simulink library "environment"  (R2024a)
settings: Solver=VariableStepAuto  StartTime=0.0  StopTime=10.0  RelTol=1e-3
undefined symbols (not defined in the file or in its folder): Heigth_brick, Heigth_ramp, Heigth_wall, Length_brick, Length_ramp, Length_wall, theta, Wall1, Wall2, Wall3, Wall4, Wall5, Wall6, Width_brick, Width_ramp, Width_wall, X, Y, Z
libraries: sm_lib x81, nesl_utility x28, $bdroot x5
(part 2 of 2)

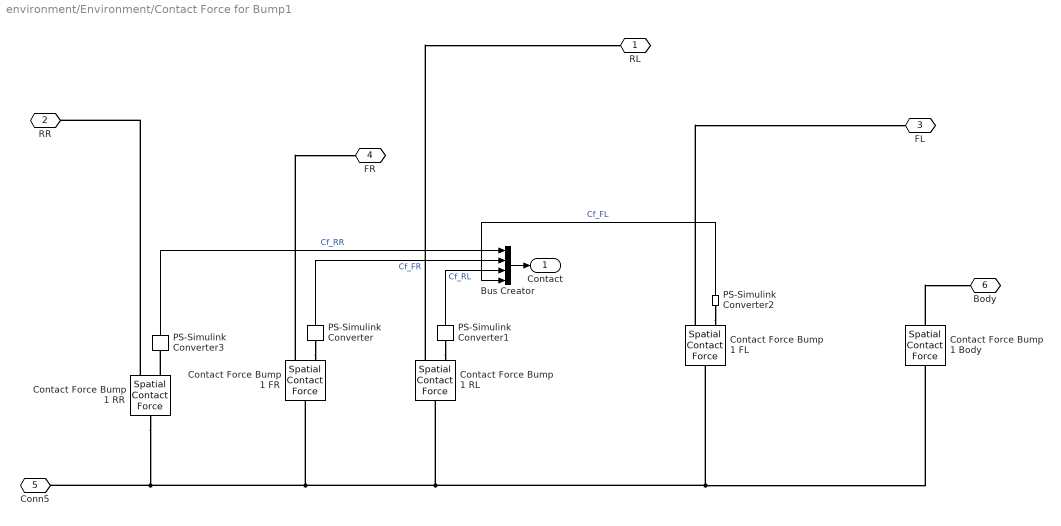
== system environment/Environment/Contact Force for Bump1 ==
  Bus Creator : BusCreator  Inputs=4
  Contact Force Bump 1 Body : sm_lib/Forces and Torques/Spatial Contact Force  NormalForceType=SmoothSpringDamper  NormalStiffness=Stiffnesscoefficient  NormalStiffnessUnits=N/m  NormalDamping=Damping_Factor  NormalDampingUnits=N/(m/s)  NormalTransitionRegionWidth=Transition_Region_Width  NormalTransitionRegionWidthUnits=m  FrictionType=SmoothStickSlip  CoefficientOfStaticFriction=Static_Friction  CoefficientOfDynamicFriction=Dynamic_Friction  FrictionalCriticalVelocity=Critical_Velocity  FrictionalCriticalVelocityUnits=m/s  SenseContactSignal=off  SensePenetrationDepth=off  SenseSeparationDistance=off  SenseNormalForceMagnitude=off  SenseFrictionalForceMagnitude=off  SenseNormalVelocity=off  SenseTangentialVelocity=off  SenseContactBaseRotation=off  SenseContactBaseTranslation=off  SenseContactFollowerRotation=off  SenseContactFollowerTranslation=off  ZeroCrossDetectContactStartAndEnd=off
  Contact Force Bump 1 FL : sm_lib/Forces and Torques/Spatial Contact Force  NormalForceType=SmoothSpringDamper  NormalStiffness=Stiffnesscoefficient  NormalStiffnessUnits=N/m  NormalDamping=Damping_Factor  NormalDampingUnits=N/(m/s)  NormalTransitionRegionWidth=Transition_Region_Width  NormalTransitionRegionWidthUnits=m  FrictionType=SmoothStickSlip  CoefficientOfStaticFriction=Static_Friction  CoefficientOfDynamicFriction=Dynamic_Friction  FrictionalCriticalVelocity=Critical_Velocity  FrictionalCriticalVelocityUnits=m/s  SenseContactSignal=off  SensePenetrationDepth=off  SenseSeparationDistance=off  SenseNormalForceMagnitude=on  SenseFrictionalForceMagnitude=off  SenseNormalVelocity=off  SenseTangentialVelocity=off  SenseContactBaseRotation=off  SenseContactBaseTranslation=off  SenseContactFollowerRotation=off  SenseContactFollowerTranslation=off  ZeroCrossDetectContactStartAndEnd=off
  Contact Force Bump 1 FR : sm_lib/Forces and Torques/Spatial Contact Force  NormalForceType=SmoothSpringDamper  NormalStiffness=Stiffnesscoefficient  NormalStiffnessUnits=N/m  NormalDamping=Damping_Factor  NormalDampingUnits=N/(m/s)  NormalTransitionRegionWidth=Transition_Region_Width  NormalTransitionRegionWidthUnits=m  FrictionType=SmoothStickSlip  CoefficientOfStaticFriction=Static_Friction  CoefficientOfDynamicFriction=Dynamic_Friction  FrictionalCriticalVelocity=Critical_Velocity  FrictionalCriticalVelocityUnits=m/s  SenseContactSignal=off  SensePenetrationDepth=off  SenseSeparationDistance=off  SenseNormalForceMagnitude=on  SenseFrictionalForceMagnitude=off  SenseNormalVelocity=off  SenseTangentialVelocity=off  SenseContactBaseRotation=off  SenseContactBaseTranslation=off  SenseContactFollowerRotation=off  SenseContactFollowerTranslation=off  ZeroCrossDetectContactStartAndEnd=off
  Contact Force Bump 1 RL : sm_lib/Forces and Torques/Spatial Contact Force  NormalForceType=SmoothSpringDamper  NormalStiffness=Stiffnesscoefficient  NormalStiffnessUnits=N/m  NormalDamping=Damping_Factor  NormalDampingUnits=N/(m/s)  NormalTransitionRegionWidth=Transition_Region_Width  NormalTransitionRegionWidthUnits=m  FrictionType=SmoothStickSlip  CoefficientOfStaticFriction=Static_Friction  CoefficientOfDynamicFriction=Dynamic_Friction  FrictionalCriticalVelocity=Critical_Velocity  FrictionalCriticalVelocityUnits=m/s  SenseContactSignal=off  SensePenetrationDepth=off  SenseSeparationDistance=off  SenseNormalForceMagnitude=on  SenseFrictionalForceMagnitude=off  SenseNormalVelocity=off  SenseTangentialVelocity=off  SenseContactBaseRotation=off  SenseContactBaseTranslation=off  SenseContactFollowerRotation=off  SenseContactFollowerTranslation=off  ZeroCrossDetectContactStartAndEnd=off
  Contact Force Bump 1 RR : sm_lib/Forces and Torques/Spatial Contact Force  NormalForceType=SmoothSpringDamper  NormalStiffness=Stiffnesscoefficient  NormalStiffnessUnits=N/m  NormalDamping=Damping_Factor  NormalDampingUnits=N/(m/s)  NormalTransitionRegionWidth=Transition_Region_Width  NormalTransitionRegionWidthUnits=m  FrictionType=SmoothStickSlip  CoefficientOfStaticFriction=Static_Friction  CoefficientOfDynamicFriction=Dynamic_Friction  FrictionalCriticalVelocity=Critical_Velocity  FrictionalCriticalVelocityUnits=m/s  SenseContactSignal=off  SensePenetrationDepth=off  SenseSeparationDistance=off  SenseNormalForceMagnitude=on  SenseFrictionalForceMagnitude=off  SenseNormalVelocity=off  SenseTangentialVelocity=off  SenseContactBaseRotation=off  SenseContactBaseTranslation=off  SenseContactFollowerRotation=off  SenseContactFollowerTranslation=off  ZeroCrossDetectContactStartAndEnd=off
  PS-Simulink Converter{,1..3} (4 alike) : nesl_utility/PS-Simulink Converter  PhysicalDomain=network_engine_domain  SubClassName=ps_output  LeftPortType=input  RightPortType=output  PseudoPeriodic=off  Frequencies=[]  VectorFormat=inherit  Unit=inherit  AffineConversion=off
  RL : PMIOPort  Side=Right
  RR : PMIOPort  Port=2  Side=Right
  FL : PMIOPort  Port=3  Side=Right
  FR : PMIOPort  Port=4  Side=Right
  Conn5 : PMIOPort  Port=5  Side=Left
  Body : PMIOPort  Port=6  Side=Right
  Contact : Outport
  wires:
  PS-Simulink Converter3/1 -> Bus Creator/1  "Cf_RR"
  PS-Simulink Converter/1 -> Bus Creator/2  "Cf_FR"
  PS-Simulink Converter1/1 -> Bus Creator/3  "Cf_RL"
  PS-Simulink Converter2/1 -> Bus Creator/4  "Cf_FL"
  Bus Creator/1 -> Contact/1
  connections:
  Contact Force Bump 1 RL/LConn1 -- Contact Force Bump 1 FR/LConn1 -- Contact Force Bump 1 RR/LConn1 -- Conn5/RConn1 -- Contact Force Bump 1 FL/LConn1 -- Contact Force Bump 1 Body/LConn1
  Contact Force Bump 1 FR/RConn1 -- FR/RConn1
  Contact Force Bump 1 RL/RConn1 -- RL/RConn1
  Contact Force Bump 1 RR/RConn1 -- RR/RConn1
  Contact Force Bump 1 FL/RConn1 -- FL/RConn1
  Contact Force Bump 1 Body/RConn1 -- Body/RConn1
  PS-Simulink Converter/LConn1 -- Contact Force Bump 1 FR/RConn2
  PS-Simulink Converter1/LConn1 -- Contact Force Bump 1 RL/RConn2
  PS-Simulink Converter2/LConn1 -- Contact Force Bump 1 FL/RConn2
  Contact Force Bump 1 RR/RConn2 -- PS-Simulink Converter3/LConn1

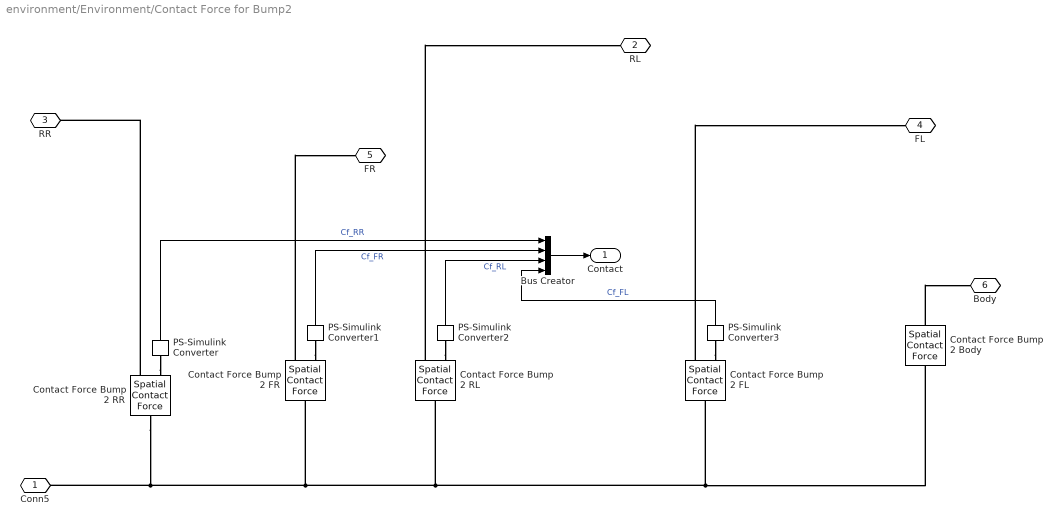
== system environment/Environment/Contact Force for Bump2 ==
  Bus Creator : BusCreator  Inputs=4
  Contact Force Bump 2 Body : sm_lib/Forces and Torques/Spatial Contact Force  NormalForceType=SmoothSpringDamper  NormalStiffness=Stiffnesscoefficient  NormalStiffnessUnits=N/m  NormalDamping=Damping_Factor  NormalDampingUnits=N/(m/s)  NormalTransitionRegionWidth=Transition_Region_Width  NormalTransitionRegionWidthUnits=m  FrictionType=SmoothStickSlip  CoefficientOfStaticFriction=Static_Friction  CoefficientOfDynamicFriction=Dynamic_Friction  FrictionalCriticalVelocity=Critical_Velocity  FrictionalCriticalVelocityUnits=m/s  SenseContactSignal=off  SensePenetrationDepth=off  SenseSeparationDistance=off  SenseNormalForceMagnitude=off  SenseFrictionalForceMagnitude=off  SenseNormalVelocity=off  SenseTangentialVelocity=off  SenseContactBaseRotation=off  SenseContactBaseTranslation=off  SenseContactFollowerRotation=off  SenseContactFollowerTranslation=off  ZeroCrossDetectContactStartAndEnd=off
  Contact Force Bump 2 FL : sm_lib/Forces and Torques/Spatial Contact Force  NormalForceType=SmoothSpringDamper  NormalStiffness=Stiffnesscoefficient  NormalStiffnessUnits=N/m  NormalDamping=Damping_Factor  NormalDampingUnits=N/(m/s)  NormalTransitionRegionWidth=Transition_Region_Width  NormalTransitionRegionWidthUnits=m  FrictionType=SmoothStickSlip  CoefficientOfStaticFriction=Static_Friction  CoefficientOfDynamicFriction=Dynamic_Friction  FrictionalCriticalVelocity=Critical_Velocity  FrictionalCriticalVelocityUnits=m/s  SenseContactSignal=off  SensePenetrationDepth=off  SenseSeparationDistance=off  SenseNormalForceMagnitude=on  SenseFrictionalForceMagnitude=off  SenseNormalVelocity=off  SenseTangentialVelocity=off  SenseContactBaseRotation=off  SenseContactBaseTranslation=off  SenseContactFollowerRotation=off  SenseContactFollowerTranslation=off  ZeroCrossDetectContactStartAndEnd=off
  Contact Force Bump 2 FR : sm_lib/Forces and Torques/Spatial Contact Force  NormalForceType=SmoothSpringDamper  NormalStiffness=Stiffnesscoefficient  NormalStiffnessUnits=N/m  NormalDamping=Damping_Factor  NormalDampingUnits=N/(m/s)  NormalTransitionRegionWidth=Transition_Region_Width  NormalTransitionRegionWidthUnits=m  FrictionType=SmoothStickSlip  CoefficientOfStaticFriction=Static_Friction  CoefficientOfDynamicFriction=Dynamic_Friction  FrictionalCriticalVelocity=Critical_Velocity  FrictionalCriticalVelocityUnits=m/s  SenseContactSignal=off  SensePenetrationDepth=off  SenseSeparationDistance=off  SenseNormalForceMagnitude=on  SenseFrictionalForceMagnitude=off  SenseNormalVelocity=off  SenseTangentialVelocity=off  SenseContactBaseRotation=off  SenseContactBaseTranslation=off  SenseContactFollowerRotation=off  SenseContactFollowerTranslation=off  ZeroCrossDetectContactStartAndEnd=off
  Contact Force Bump 2 RL : sm_lib/Forces and Torques/Spatial Contact Force  NormalForceType=SmoothSpringDamper  NormalStiffness=Stiffnesscoefficient  NormalStiffnessUnits=N/m  NormalDamping=Damping_Factor  NormalDampingUnits=N/(m/s)  NormalTransitionRegionWidth=Transition_Region_Width  NormalTransitionRegionWidthUnits=m  FrictionType=SmoothStickSlip  CoefficientOfStaticFriction=Static_Friction  CoefficientOfDynamicFriction=Dynamic_Friction  FrictionalCriticalVelocity=Critical_Velocity  FrictionalCriticalVelocityUnits=m/s  SenseContactSignal=off  SensePenetrationDepth=off  SenseSeparationDistance=off  SenseNormalForceMagnitude=on  SenseFrictionalForceMagnitude=off  SenseNormalVelocity=off  SenseTangentialVelocity=off  SenseContactBaseRotation=off  SenseContactBaseTranslation=off  SenseContactFollowerRotation=off  SenseContactFollowerTranslation=off  ZeroCrossDetectContactStartAndEnd=off
  Contact Force Bump 2 RR : sm_lib/Forces and Torques/Spatial Contact Force  NormalForceType=SmoothSpringDamper  NormalStiffness=Stiffnesscoefficient  NormalStiffnessUnits=N/m  NormalDamping=Damping_Factor  NormalDampingUnits=N/(m/s)  NormalTransitionRegionWidth=Transition_Region_Width  NormalTransitionRegionWidthUnits=m  FrictionType=SmoothStickSlip  CoefficientOfStaticFriction=Static_Friction  CoefficientOfDynamicFriction=Dynamic_Friction  FrictionalCriticalVelocity=Critical_Velocity  FrictionalCriticalVelocityUnits=m/s  SenseContactSignal=off  SensePenetrationDepth=off  SenseSeparationDistance=off  SenseNormalForceMagnitude=on  SenseFrictionalForceMagnitude=off  SenseNormalVelocity=off  SenseTangentialVelocity=off  SenseContactBaseRotation=off  SenseContactBaseTranslation=off  SenseContactFollowerRotation=off  SenseContactFollowerTranslation=off  ZeroCrossDetectContactStartAndEnd=off
  PS-Simulink Converter{,1..3} (4 alike) : nesl_utility/PS-Simulink Converter  PhysicalDomain=network_engine_domain  SubClassName=ps_output  LeftPortType=input  RightPortType=output  PseudoPeriodic=off  Frequencies=[]  VectorFormat=inherit  Unit=inherit  AffineConversion=off
  Conn5 : PMIOPort  Side=Left
  RL : PMIOPort  Port=2  Side=Right
  RR : PMIOPort  Port=3  Side=Right
  FL : PMIOPort  Port=4  Side=Right
  FR : PMIOPort  Port=5  Side=Right
  Body : PMIOPort  Port=6  Side=Right
  Contact : Outport
  wires:
  PS-Simulink Converter/1 -> Bus Creator/1  "Cf_RR"
  PS-Simulink Converter1/1 -> Bus Creator/2  "Cf_FR"
  PS-Simulink Converter2/1 -> Bus Creator/3  "Cf_RL"
  PS-Simulink Converter3/1 -> Bus Creator/4  "Cf_FL"
  Bus Creator/1 -> Contact/1
  connections:
  Contact Force Bump 2 RL/LConn1 -- Contact Force Bump 2 FR/LConn1 -- Contact Force Bump 2 RR/LConn1 -- Conn5/RConn1 -- Contact Force Bump 2 FL/LConn1 -- Contact Force Bump 2 Body/LConn1
  Contact Force Bump 2 FR/RConn1 -- FR/RConn1
  Contact Force Bump 2 RL/RConn1 -- RL/RConn1
  Contact Force Bump 2 RR/RConn1 -- RR/RConn1
  Contact Force Bump 2 FL/RConn1 -- FL/RConn1
  Contact Force Bump 2 Body/RConn1 -- Body/RConn1
  PS-Simulink Converter/LConn1 -- Contact Force Bump 2 RR/RConn2
  PS-Simulink Converter1/LConn1 -- Contact Force Bump 2 FR/RConn2
  PS-Simulink Converter2/LConn1 -- Contact Force Bump 2 RL/RConn2
  PS-Simulink Converter3/LConn1 -- Contact Force Bump 2 FL/RConn2

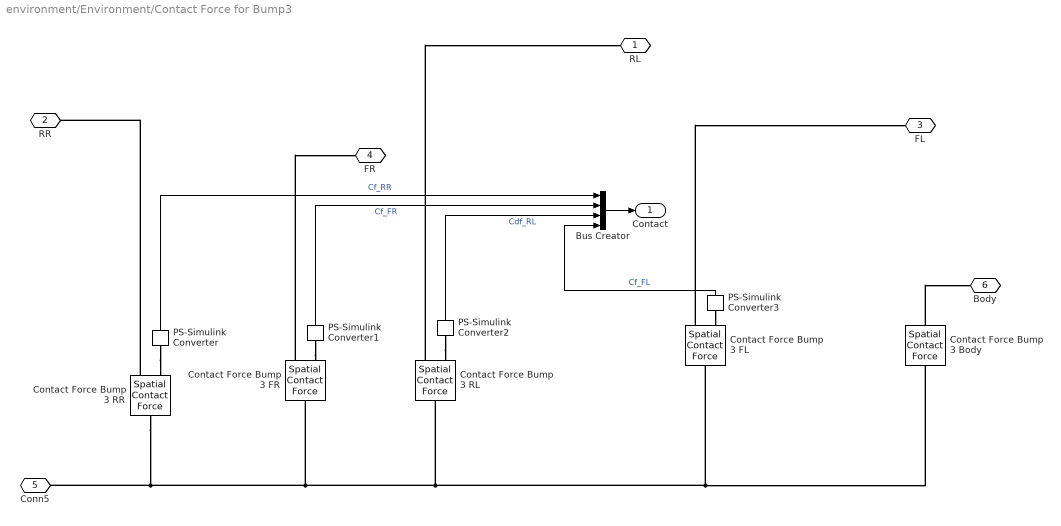
== system environment/Environment/Contact Force for Bump3 ==
  Bus Creator : BusCreator  Inputs=4
  Contact Force Bump 3 Body : sm_lib/Forces and Torques/Spatial Contact Force  NormalForceType=SmoothSpringDamper  NormalStiffness=Stiffnesscoefficient  NormalStiffnessUnits=N/m  NormalDamping=Damping_Factor  NormalDampingUnits=N/(m/s)  NormalTransitionRegionWidth=Transition_Region_Width  NormalTransitionRegionWidthUnits=m  FrictionType=SmoothStickSlip  CoefficientOfStaticFriction=Static_Friction  CoefficientOfDynamicFriction=Dynamic_Friction  FrictionalCriticalVelocity=Critical_Velocity  FrictionalCriticalVelocityUnits=m/s  SenseContactSignal=off  SensePenetrationDepth=off  SenseSeparationDistance=off  SenseNormalForceMagnitude=off  SenseFrictionalForceMagnitude=off  SenseNormalVelocity=off  SenseTangentialVelocity=off  SenseContactBaseRotation=off  SenseContactBaseTranslation=off  SenseContactFollowerRotation=off  SenseContactFollowerTranslation=off  ZeroCrossDetectContactStartAndEnd=off
  Contact Force Bump 3 FL : sm_lib/Forces and Torques/Spatial Contact Force  NormalForceType=SmoothSpringDamper  NormalStiffness=Stiffnesscoefficient  NormalStiffnessUnits=N/m  NormalDamping=Damping_Factor  NormalDampingUnits=N/(m/s)  NormalTransitionRegionWidth=Transition_Region_Width  NormalTransitionRegionWidthUnits=m  FrictionType=SmoothStickSlip  CoefficientOfStaticFriction=Static_Friction  CoefficientOfDynamicFriction=Dynamic_Friction  FrictionalCriticalVelocity=Critical_Velocity  FrictionalCriticalVelocityUnits=m/s  SenseContactSignal=off  SensePenetrationDepth=off  SenseSeparationDistance=off  SenseNormalForceMagnitude=on  SenseFrictionalForceMagnitude=off  SenseNormalVelocity=off  SenseTangentialVelocity=off  SenseContactBaseRotation=off  SenseContactBaseTranslation=off  SenseContactFollowerRotation=off  SenseContactFollowerTranslation=off  ZeroCrossDetectContactStartAndEnd=off
  Contact Force Bump 3 FR : sm_lib/Forces and Torques/Spatial Contact Force  NormalForceType=SmoothSpringDamper  NormalStiffness=Stiffnesscoefficient  NormalStiffnessUnits=N/m  NormalDamping=Damping_Factor  NormalDampingUnits=N/(m/s)  NormalTransitionRegionWidth=Transition_Region_Width  NormalTransitionRegionWidthUnits=m  FrictionType=SmoothStickSlip  CoefficientOfStaticFriction=Static_Friction  CoefficientOfDynamicFriction=Dynamic_Friction  FrictionalCriticalVelocity=Critical_Velocity  FrictionalCriticalVelocityUnits=m/s  SenseContactSignal=off  SensePenetrationDepth=off  SenseSeparationDistance=off  SenseNormalForceMagnitude=on  SenseFrictionalForceMagnitude=off  SenseNormalVelocity=off  SenseTangentialVelocity=off  SenseContactBaseRotation=off  SenseContactBaseTranslation=off  SenseContactFollowerRotation=off  SenseContactFollowerTranslation=off  ZeroCrossDetectContactStartAndEnd=off
  Contact Force Bump 3 RL : sm_lib/Forces and Torques/Spatial Contact Force  NormalForceType=SmoothSpringDamper  NormalStiffness=Stiffnesscoefficient  NormalStiffnessUnits=N/m  NormalDamping=Damping_Factor  NormalDampingUnits=N/(m/s)  NormalTransitionRegionWidth=Transition_Region_Width  NormalTransitionRegionWidthUnits=m  FrictionType=SmoothStickSlip  CoefficientOfStaticFriction=Static_Friction  CoefficientOfDynamicFriction=Dynamic_Friction  FrictionalCriticalVelocity=Critical_Velocity  FrictionalCriticalVelocityUnits=m/s  SenseContactSignal=off  SensePenetrationDepth=off  SenseSeparationDistance=off  SenseNormalForceMagnitude=on  SenseFrictionalForceMagnitude=off  SenseNormalVelocity=off  SenseTangentialVelocity=off  SenseContactBaseRotation=off  SenseContactBaseTranslation=off  SenseContactFollowerRotation=off  SenseContactFollowerTranslation=off  ZeroCrossDetectContactStartAndEnd=off
  Contact Force Bump 3 RR : sm_lib/Forces and Torques/Spatial Contact Force  NormalForceType=SmoothSpringDamper  NormalStiffness=Stiffnesscoefficient  NormalStiffnessUnits=N/m  NormalDamping=Damping_Factor  NormalDampingUnits=N/(m/s)  NormalTransitionRegionWidth=Transition_Region_Width  NormalTransitionRegionWidthUnits=m  FrictionType=SmoothStickSlip  CoefficientOfStaticFriction=Static_Friction  CoefficientOfDynamicFriction=Dynamic_Friction  FrictionalCriticalVelocity=Critical_Velocity  FrictionalCriticalVelocityUnits=m/s  SenseContactSignal=off  SensePenetrationDepth=off  SenseSeparationDistance=off  SenseNormalForceMagnitude=on  SenseFrictionalForceMagnitude=off  SenseNormalVelocity=off  SenseTangentialVelocity=off  SenseContactBaseRotation=off  SenseContactBaseTranslation=off  SenseContactFollowerRotation=off  SenseContactFollowerTranslation=off  ZeroCrossDetectContactStartAndEnd=off
  PS-Simulink Converter{,1..3} (4 alike) : nesl_utility/PS-Simulink Converter  PhysicalDomain=network_engine_domain  SubClassName=ps_output  LeftPortType=input  RightPortType=output  PseudoPeriodic=off  Frequencies=[]  VectorFormat=inherit  Unit=inherit  AffineConversion=off
  RL : PMIOPort  Side=Right
  RR : PMIOPort  Port=2  Side=Right
  FL : PMIOPort  Port=3  Side=Right
  FR : PMIOPort  Port=4  Side=Right
  Conn5 : PMIOPort  Port=5  Side=Left
  Body : PMIOPort  Port=6  Side=Right
  Contact : Outport
  wires:
  PS-Simulink Converter/1 -> Bus Creator/1  "Cf_RR"
  PS-Simulink Converter1/1 -> Bus Creator/2  "Cf_FR"
  PS-Simulink Converter2/1 -> Bus Creator/3  "Cdf_RL"
  PS-Simulink Converter3/1 -> Bus Creator/4  "Cf_FL"
  Bus Creator/1 -> Contact/1
  connections:
  Contact Force Bump 3 RL/LConn1 -- Contact Force Bump 3 FR/LConn1 -- Contact Force Bump 3 RR/LConn1 -- Conn5/RConn1 -- Contact Force Bump 3 FL/LConn1 -- Contact Force Bump 3 Body/LConn1
  Contact Force Bump 3 FR/RConn1 -- FR/RConn1
  Contact Force Bump 3 RL/RConn1 -- RL/RConn1
  Contact Force Bump 3 RR/RConn1 -- RR/RConn1
  Contact Force Bump 3 FL/RConn1 -- FL/RConn1
  Contact Force Bump 3 Body/RConn1 -- Body/RConn1
  PS-Simulink Converter/LConn1 -- Contact Force Bump 3 RR/RConn2
  PS-Simulink Converter1/LConn1 -- Contact Force Bump 3 FR/RConn2
  PS-Simulink Converter2/LConn1 -- Contact Force Bump 3 RL/RConn2
  PS-Simulink Converter3/LConn1 -- Contact Force Bump 3 FL/RConn2

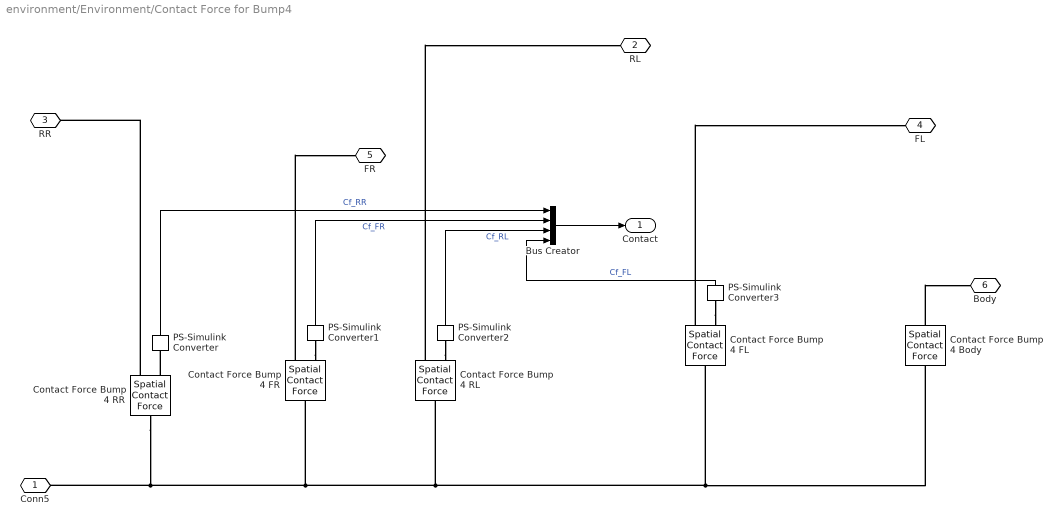
== system environment/Environment/Contact Force for Bump4 ==
  Bus Creator : BusCreator  Inputs=4
  Contact Force Bump 4 Body : sm_lib/Forces and Torques/Spatial Contact Force  NormalForceType=SmoothSpringDamper  NormalStiffness=Stiffnesscoefficient  NormalStiffnessUnits=N/m  NormalDamping=Damping_Factor  NormalDampingUnits=N/(m/s)  NormalTransitionRegionWidth=Transition_Region_Width  NormalTransitionRegionWidthUnits=m  FrictionType=SmoothStickSlip  CoefficientOfStaticFriction=Static_Friction  CoefficientOfDynamicFriction=Dynamic_Friction  FrictionalCriticalVelocity=Critical_Velocity  FrictionalCriticalVelocityUnits=m/s  SenseContactSignal=off  SensePenetrationDepth=off  SenseSeparationDistance=off  SenseNormalForceMagnitude=off  SenseFrictionalForceMagnitude=off  SenseNormalVelocity=off  SenseTangentialVelocity=off  SenseContactBaseRotation=off  SenseContactBaseTranslation=off  SenseContactFollowerRotation=off  SenseContactFollowerTranslation=off  ZeroCrossDetectContactStartAndEnd=off
  Contact Force Bump 4 FL : sm_lib/Forces and Torques/Spatial Contact Force  NormalForceType=SmoothSpringDamper  NormalStiffness=Stiffnesscoefficient  NormalStiffnessUnits=N/m  NormalDamping=Damping_Factor  NormalDampingUnits=N/(m/s)  NormalTransitionRegionWidth=Transition_Region_Width  NormalTransitionRegionWidthUnits=m  FrictionType=SmoothStickSlip  CoefficientOfStaticFriction=Static_Friction  CoefficientOfDynamicFriction=Dynamic_Friction  FrictionalCriticalVelocity=Critical_Velocity  FrictionalCriticalVelocityUnits=m/s  SenseContactSignal=off  SensePenetrationDepth=off  SenseSeparationDistance=off  SenseNormalForceMagnitude=on  SenseFrictionalForceMagnitude=off  SenseNormalVelocity=off  SenseTangentialVelocity=off  SenseContactBaseRotation=off  SenseContactBaseTranslation=off  SenseContactFollowerRotation=off  SenseContactFollowerTranslation=off  ZeroCrossDetectContactStartAndEnd=off
  Contact Force Bump 4 FR : sm_lib/Forces and Torques/Spatial Contact Force  NormalForceType=SmoothSpringDamper  NormalStiffness=Stiffnesscoefficient  NormalStiffnessUnits=N/m  NormalDamping=Damping_Factor  NormalDampingUnits=N/(m/s)  NormalTransitionRegionWidth=Transition_Region_Width  NormalTransitionRegionWidthUnits=m  FrictionType=SmoothStickSlip  CoefficientOfStaticFriction=Static_Friction  CoefficientOfDynamicFriction=Dynamic_Friction  FrictionalCriticalVelocity=Critical_Velocity  FrictionalCriticalVelocityUnits=m/s  SenseContactSignal=off  SensePenetrationDepth=off  SenseSeparationDistance=off  SenseNormalForceMagnitude=on  SenseFrictionalForceMagnitude=off  SenseNormalVelocity=off  SenseTangentialVelocity=off  SenseContactBaseRotation=off  SenseContactBaseTranslation=off  SenseContactFollowerRotation=off  SenseContactFollowerTranslation=off  ZeroCrossDetectContactStartAndEnd=off
  Contact Force Bump 4 RL : sm_lib/Forces and Torques/Spatial Contact Force  NormalForceType=SmoothSpringDamper  NormalStiffness=Stiffnesscoefficient  NormalStiffnessUnits=N/m  NormalDamping=Damping_Factor  NormalDampingUnits=N/(m/s)  NormalTransitionRegionWidth=Transition_Region_Width  NormalTransitionRegionWidthUnits=m  FrictionType=SmoothStickSlip  CoefficientOfStaticFriction=Static_Friction  CoefficientOfDynamicFriction=Dynamic_Friction  FrictionalCriticalVelocity=Critical_Velocity  FrictionalCriticalVelocityUnits=m/s  SenseContactSignal=off  SensePenetrationDepth=off  SenseSeparationDistance=off  SenseNormalForceMagnitude=on  SenseFrictionalForceMagnitude=off  SenseNormalVelocity=off  SenseTangentialVelocity=off  SenseContactBaseRotation=off  SenseContactBaseTranslation=off  SenseContactFollowerRotation=off  SenseContactFollowerTranslation=off  ZeroCrossDetectContactStartAndEnd=off
  Contact Force Bump 4 RR : sm_lib/Forces and Torques/Spatial Contact Force  NormalForceType=SmoothSpringDamper  NormalStiffness=Stiffnesscoefficient  NormalStiffnessUnits=N/m  NormalDamping=Damping_Factor  NormalDampingUnits=N/(m/s)  NormalTransitionRegionWidth=Transition_Region_Width  NormalTransitionRegionWidthUnits=m  FrictionType=SmoothStickSlip  CoefficientOfStaticFriction=Static_Friction  CoefficientOfDynamicFriction=Dynamic_Friction  FrictionalCriticalVelocity=Critical_Velocity  FrictionalCriticalVelocityUnits=m/s  SenseContactSignal=off  SensePenetrationDepth=off  SenseSeparationDistance=off  SenseNormalForceMagnitude=on  SenseFrictionalForceMagnitude=off  SenseNormalVelocity=off  SenseTangentialVelocity=off  SenseContactBaseRotation=off  SenseContactBaseTranslation=off  SenseContactFollowerRotation=off  SenseContactFollowerTranslation=off  ZeroCrossDetectContactStartAndEnd=off
  PS-Simulink Converter{,1..3} (4 alike) : nesl_utility/PS-Simulink Converter  PhysicalDomain=network_engine_domain  SubClassName=ps_output  LeftPortType=input  RightPortType=output  PseudoPeriodic=off  Frequencies=[]  VectorFormat=inherit  Unit=inherit  AffineConversion=off
  Conn5 : PMIOPort  Side=Left
  RL : PMIOPort  Port=2  Side=Right
  RR : PMIOPort  Port=3  Side=Right
  FL : PMIOPort  Port=4  Side=Right
  FR : PMIOPort  Port=5  Side=Right
  Body : PMIOPort  Port=6  Side=Right
  Contact : Outport
  wires:
  Bus Creator/1 -> Contact/1
  PS-Simulink Converter/1 -> Bus Creator/1  "Cf_RR"
  PS-Simulink Converter1/1 -> Bus Creator/2  "Cf_FR"
  PS-Simulink Converter2/1 -> Bus Creator/3  "Cf_RL"
  PS-Simulink Converter3/1 -> Bus Creator/4  "Cf_FL"
  connections:
  Contact Force Bump 4 RL/LConn1 -- Contact Force Bump 4 FR/LConn1 -- Contact Force Bump 4 RR/LConn1 -- Conn5/RConn1 -- Contact Force Bump 4 FL/LConn1 -- Contact Force Bump 4 Body/LConn1
  Contact Force Bump 4 FR/RConn1 -- FR/RConn1
  Contact Force Bump 4 RL/RConn1 -- RL/RConn1
  Contact Force Bump 4 RR/RConn1 -- RR/RConn1
  Contact Force Bump 4 FL/RConn1 -- FL/RConn1
  Contact Force Bump 4 Body/RConn1 -- Body/RConn1
  Contact Force Bump 4 RR/RConn2 -- PS-Simulink Converter/LConn1
  PS-Simulink Converter1/LConn1 -- Contact Force Bump 4 FR/RConn2
  PS-Simulink Converter2/LConn1 -- Contact Force Bump 4 RL/RConn2
  PS-Simulink Converter3/LConn1 -- Contact Force Bump 4 FL/RConn2

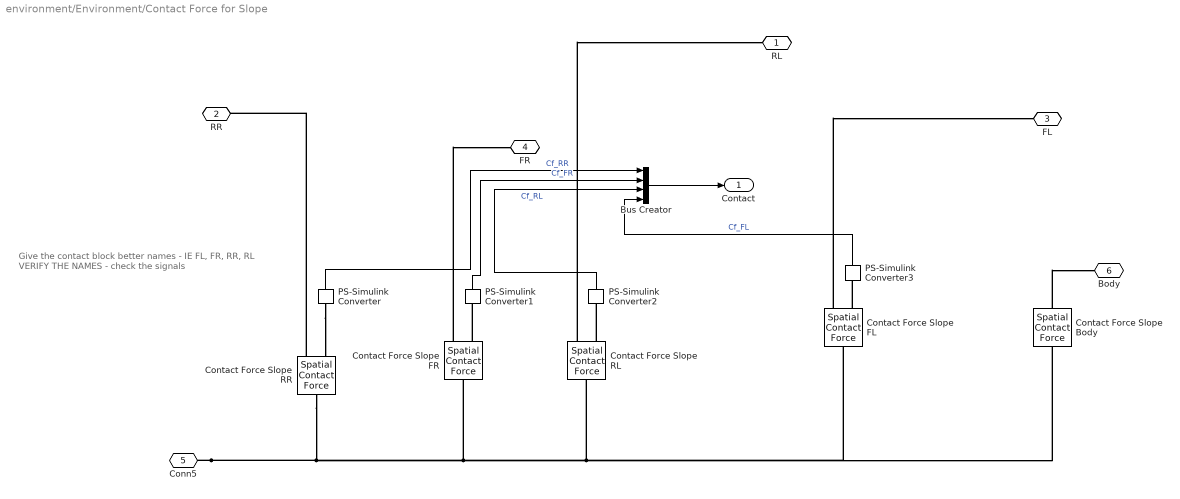
== system environment/Environment/Contact Force for Slope ==
  note: Give the contact block better names - IE FL, FR, RR, RL
      | VERIFY THE NAMES - check the signals
  Bus Creator : BusCreator  Inputs=4
  Contact Force Slope Body : sm_lib/Forces and Torques/Spatial Contact Force  NormalForceType=SmoothSpringDamper  NormalStiffness=Stiffnesscoefficient  NormalStiffnessUnits=N/m  NormalDamping=Damping_Factor  NormalDampingUnits=N/(m/s)  NormalTransitionRegionWidth=Transition_Region_Width  NormalTransitionRegionWidthUnits=m  FrictionType=SmoothStickSlip  CoefficientOfStaticFriction=Static_Friction  CoefficientOfDynamicFriction=Dynamic_Friction  FrictionalCriticalVelocity=Critical_Velocity  FrictionalCriticalVelocityUnits=m/s  SenseContactSignal=off  SensePenetrationDepth=off  SenseSeparationDistance=off  SenseNormalForceMagnitude=off  SenseFrictionalForceMagnitude=off  SenseNormalVelocity=off  SenseTangentialVelocity=off  SenseContactBaseRotation=off  SenseContactBaseTranslation=off  SenseContactFollowerRotation=off  SenseContactFollowerTranslation=off  ZeroCrossDetectContactStartAndEnd=off
  Contact Force Slope FL : sm_lib/Forces and Torques/Spatial Contact Force  NormalForceType=SmoothSpringDamper  NormalStiffness=Stiffnesscoefficient  NormalStiffnessUnits=N/m  NormalDamping=Damping_Factor  NormalDampingUnits=N/(m/s)  NormalTransitionRegionWidth=Transition_Region_Width  NormalTransitionRegionWidthUnits=m  FrictionType=SmoothStickSlip  CoefficientOfStaticFriction=Static_Friction  CoefficientOfDynamicFriction=Dynamic_Friction  FrictionalCriticalVelocity=Critical_Velocity  FrictionalCriticalVelocityUnits=m/s  SenseContactSignal=off  SensePenetrationDepth=off  SenseSeparationDistance=off  SenseNormalForceMagnitude=on  SenseFrictionalForceMagnitude=off  SenseNormalVelocity=off  SenseTangentialVelocity=off  SenseContactBaseRotation=off  SenseContactBaseTranslation=off  SenseContactFollowerRotation=off  SenseContactFollowerTranslation=off  ZeroCrossDetectContactStartAndEnd=off
  Contact Force Slope FR : sm_lib/Forces and Torques/Spatial Contact Force  NormalForceType=SmoothSpringDamper  NormalStiffness=Stiffnesscoefficient  NormalStiffnessUnits=N/m  NormalDamping=Damping_Factor  NormalDampingUnits=N/(m/s)  NormalTransitionRegionWidth=Transition_Region_Width  NormalTransitionRegionWidthUnits=m  FrictionType=SmoothStickSlip  CoefficientOfStaticFriction=Static_Friction  CoefficientOfDynamicFriction=Dynamic_Friction  FrictionalCriticalVelocity=Critical_Velocity  FrictionalCriticalVelocityUnits=m/s  SenseContactSignal=off  SensePenetrationDepth=off  SenseSeparationDistance=off  SenseNormalForceMagnitude=on  SenseFrictionalForceMagnitude=off  SenseNormalVelocity=off  SenseTangentialVelocity=off  SenseContactBaseRotation=off  SenseContactBaseTranslation=off  SenseContactFollowerRotation=off  SenseContactFollowerTranslation=off  ZeroCrossDetectContactStartAndEnd=off
  Contact Force Slope RL : sm_lib/Forces and Torques/Spatial Contact Force  NormalForceType=SmoothSpringDamper  NormalStiffness=Stiffnesscoefficient  NormalStiffnessUnits=N/m  NormalDamping=Damping_Factor  NormalDampingUnits=N/(m/s)  NormalTransitionRegionWidth=Transition_Region_Width  NormalTransitionRegionWidthUnits=m  FrictionType=SmoothStickSlip  CoefficientOfStaticFriction=Static_Friction  CoefficientOfDynamicFriction=Dynamic_Friction  FrictionalCriticalVelocity=Critical_Velocity  FrictionalCriticalVelocityUnits=m/s  SenseContactSignal=off  SensePenetrationDepth=off  SenseSeparationDistance=off  SenseNormalForceMagnitude=on  SenseFrictionalForceMagnitude=off  SenseNormalVelocity=off  SenseTangentialVelocity=off  SenseContactBaseRotation=off  SenseContactBaseTranslation=off  SenseContactFollowerRotation=off  SenseContactFollowerTranslation=off  ZeroCrossDetectContactStartAndEnd=off
  Contact Force Slope RR : sm_lib/Forces and Torques/Spatial Contact Force  NormalForceType=SmoothSpringDamper  NormalStiffness=Stiffnesscoefficient  NormalStiffnessUnits=N/m  NormalDamping=Damping_Factor  NormalDampingUnits=N/(m/s)  NormalTransitionRegionWidth=Transition_Region_Width  NormalTransitionRegionWidthUnits=m  FrictionType=SmoothStickSlip  CoefficientOfStaticFriction=Static_Friction  CoefficientOfDynamicFriction=Dynamic_Friction  FrictionalCriticalVelocity=Critical_Velocity  FrictionalCriticalVelocityUnits=m/s  SenseContactSignal=off  SensePenetrationDepth=off  SenseSeparationDistance=off  SenseNormalForceMagnitude=on  SenseFrictionalForceMagnitude=off  SenseNormalVelocity=off  SenseTangentialVelocity=off  SenseContactBaseRotation=off  SenseContactBaseTranslation=off  SenseContactFollowerRotation=off  SenseContactFollowerTranslation=off  ZeroCrossDetectContactStartAndEnd=off
  PS-Simulink Converter{,1..3} (4 alike) : nesl_utility/PS-Simulink Converter  PhysicalDomain=network_engine_domain  SubClassName=ps_output  LeftPortType=input  RightPortType=output  PseudoPeriodic=off  Frequencies=[]  VectorFormat=inherit  Unit=inherit  AffineConversion=off
  RL : PMIOPort  Side=Right
  RR : PMIOPort  Port=2  Side=Right
  FL : PMIOPort  Port=3  Side=Right
  FR : PMIOPort  Port=4  Side=Right
  Conn5 : PMIOPort  Port=5  Side=Left
  Body : PMIOPort  Port=6  Side=Right
  Contact : Outport
  wires:
  Bus Creator/1 -> Contact/1
  PS-Simulink Converter3/1 -> Bus Creator/4  "Cf_FL"
  PS-Simulink Converter2/1 -> Bus Creator/3  "Cf_RL"
  PS-Simulink Converter1/1 -> Bus Creator/2  "Cf_FR"
  PS-Simulink Converter/1 -> Bus Creator/1  "Cf_RR"
  connections:
  Contact Force Slope RL/RConn2 -- PS-Simulink Converter2/LConn1
  Contact Force Slope FL/RConn2 -- PS-Simulink Converter3/LConn1
  Contact Force Slope FR/RConn2 -- PS-Simulink Converter1/LConn1
  PS-Simulink Converter/LConn1 -- Contact Force Slope RR/RConn2
  Contact Force Slope Body/RConn1 -- Body/RConn1
  Contact Force Slope FL/RConn1 -- FL/RConn1
  Contact Force Slope RR/RConn1 -- RR/RConn1
  Contact Force Slope RL/RConn1 -- RL/RConn1
  Contact Force Slope FR/RConn1 -- FR/RConn1
  Conn5/RConn1 -- Contact Force Slope FR/LConn1 -- Contact Force Slope RL/LConn1 -- Contact Force Slope FL/LConn1 -- Contact Force Slope Body/LConn1 -- Contact Force Slope RR/LConn1

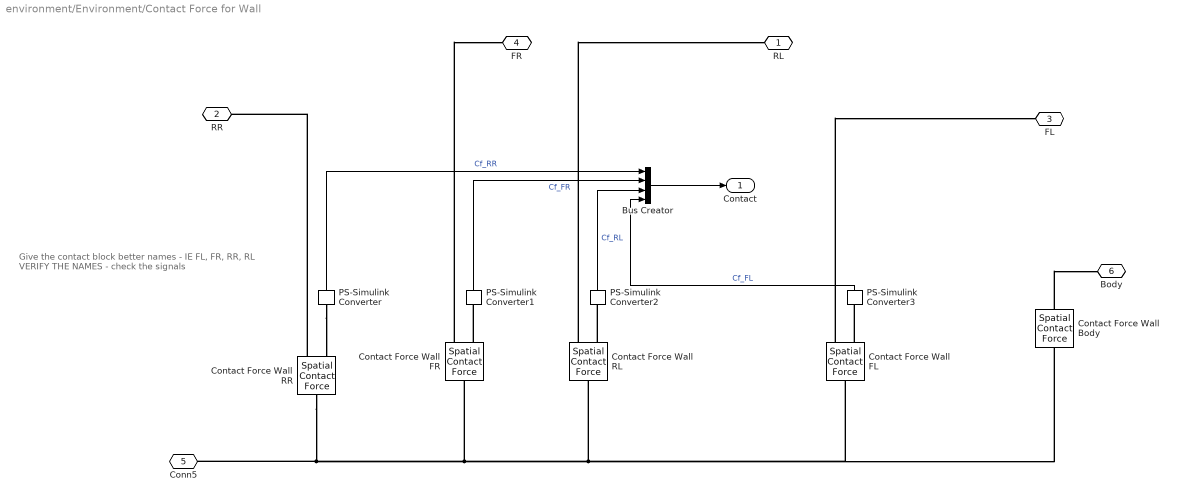
== system environment/Environment/Contact Force for Wall ==
  note: Give the contact block better names - IE FL, FR, RR, RL
      | VERIFY THE NAMES - check the signals
  Bus Creator : BusCreator  Inputs=4
  Contact Force Wall Body : sm_lib/Forces and Torques/Spatial Contact Force  NormalForceType=SmoothSpringDamper  NormalStiffness=Stiffnesscoefficient  NormalStiffnessUnits=N/m  NormalDamping=Damping_Factor  NormalDampingUnits=N/(m/s)  NormalTransitionRegionWidth=Transition_Region_Width  NormalTransitionRegionWidthUnits=m  FrictionType=SmoothStickSlip  CoefficientOfStaticFriction=Static_Friction  CoefficientOfDynamicFriction=Dynamic_Friction  FrictionalCriticalVelocity=Critical_Velocity  FrictionalCriticalVelocityUnits=m/s  SenseContactSignal=off  SensePenetrationDepth=off  SenseSeparationDistance=off  SenseNormalForceMagnitude=off  SenseFrictionalForceMagnitude=off  SenseNormalVelocity=off  SenseTangentialVelocity=off  SenseContactBaseRotation=off  SenseContactBaseTranslation=off  SenseContactFollowerRotation=off  SenseContactFollowerTranslation=off  ZeroCrossDetectContactStartAndEnd=off
  Contact Force Wall FL : sm_lib/Forces and Torques/Spatial Contact Force  NormalForceType=SmoothSpringDamper  NormalStiffness=Stiffnesscoefficient  NormalStiffnessUnits=N/m  NormalDamping=Damping_Factor  NormalDampingUnits=N/(m/s)  NormalTransitionRegionWidth=Transition_Region_Width  NormalTransitionRegionWidthUnits=m  FrictionType=SmoothStickSlip  CoefficientOfStaticFriction=Static_Friction  CoefficientOfDynamicFriction=Dynamic_Friction  FrictionalCriticalVelocity=Critical_Velocity  FrictionalCriticalVelocityUnits=m/s  SenseContactSignal=off  SensePenetrationDepth=off  SenseSeparationDistance=off  SenseNormalForceMagnitude=on  SenseFrictionalForceMagnitude=off  SenseNormalVelocity=off  SenseTangentialVelocity=off  SenseContactBaseRotation=off  SenseContactBaseTranslation=off  SenseContactFollowerRotation=off  SenseContactFollowerTranslation=off  ZeroCrossDetectContactStartAndEnd=off
  Contact Force Wall FR : sm_lib/Forces and Torques/Spatial Contact Force  NormalForceType=SmoothSpringDamper  NormalStiffness=Stiffnesscoefficient  NormalStiffnessUnits=N/m  NormalDamping=Damping_Factor  NormalDampingUnits=N/(m/s)  NormalTransitionRegionWidth=Transition_Region_Width  NormalTransitionRegionWidthUnits=m  FrictionType=SmoothStickSlip  CoefficientOfStaticFriction=Static_Friction  CoefficientOfDynamicFriction=Dynamic_Friction  FrictionalCriticalVelocity=Critical_Velocity  FrictionalCriticalVelocityUnits=m/s  SenseContactSignal=off  SensePenetrationDepth=off  SenseSeparationDistance=off  SenseNormalForceMagnitude=on  SenseFrictionalForceMagnitude=off  SenseNormalVelocity=off  SenseTangentialVelocity=off  SenseContactBaseRotation=off  SenseContactBaseTranslation=off  SenseContactFollowerRotation=off  SenseContactFollowerTranslation=off  ZeroCrossDetectContactStartAndEnd=off
  Contact Force Wall RL : sm_lib/Forces and Torques/Spatial Contact Force  NormalForceType=SmoothSpringDamper  NormalStiffness=Stiffnesscoefficient  NormalStiffnessUnits=N/m  NormalDamping=Damping_Factor  NormalDampingUnits=N/(m/s)  NormalTransitionRegionWidth=Transition_Region_Width  NormalTransitionRegionWidthUnits=m  FrictionType=SmoothStickSlip  CoefficientOfStaticFriction=Static_Friction  CoefficientOfDynamicFriction=Dynamic_Friction  FrictionalCriticalVelocity=Critical_Velocity  FrictionalCriticalVelocityUnits=m/s  SenseContactSignal=off  SensePenetrationDepth=off  SenseSeparationDistance=off  SenseNormalForceMagnitude=on  SenseFrictionalForceMagnitude=off  SenseNormalVelocity=off  SenseTangentialVelocity=off  SenseContactBaseRotation=off  SenseContactBaseTranslation=off  SenseContactFollowerRotation=off  SenseContactFollowerTranslation=off  ZeroCrossDetectContactStartAndEnd=off
  Contact Force Wall RR : sm_lib/Forces and Torques/Spatial Contact Force  NormalForceType=SmoothSpringDamper  NormalStiffness=Stiffnesscoefficient  NormalStiffnessUnits=N/m  NormalDamping=Damping_Factor  NormalDampingUnits=N/(m/s)  NormalTransitionRegionWidth=Transition_Region_Width  NormalTransitionRegionWidthUnits=m  FrictionType=SmoothStickSlip  CoefficientOfStaticFriction=Static_Friction  CoefficientOfDynamicFriction=Dynamic_Friction  FrictionalCriticalVelocity=Critical_Velocity  FrictionalCriticalVelocityUnits=m/s  SenseContactSignal=off  SensePenetrationDepth=off  SenseSeparationDistance=off  SenseNormalForceMagnitude=on  SenseFrictionalForceMagnitude=off  SenseNormalVelocity=off  SenseTangentialVelocity=off  SenseContactBaseRotation=off  SenseContactBaseTranslation=off  SenseContactFollowerRotation=off  SenseContactFollowerTranslation=off  ZeroCrossDetectContactStartAndEnd=off
  PS-Simulink Converter{,1..3} (4 alike) : nesl_utility/PS-Simulink Converter  PhysicalDomain=network_engine_domain  SubClassName=ps_output  LeftPortType=input  RightPortType=output  PseudoPeriodic=off  Frequencies=[]  VectorFormat=inherit  Unit=inherit  AffineConversion=off
  RL : PMIOPort  Side=Right
  RR : PMIOPort  Port=2  Side=Right
  FL : PMIOPort  Port=3  Side=Right
  FR : PMIOPort  Port=4  Side=Right
  Conn5 : PMIOPort  Port=5  Side=Left
  Body : PMIOPort  Port=6  Side=Right
  Contact : Outport
  wires:
  PS-Simulink Converter/1 -> Bus Creator/1  "Cf_RR"
  PS-Simulink Converter1/1 -> Bus Creator/2  "Cf_FR"
  PS-Simulink Converter2/1 -> Bus Creator/3  "Cf_RL"
  PS-Simulink Converter3/1 -> Bus Creator/4  "Cf_FL"
  Bus Creator/1 -> Contact/1
  connections:
  Contact Force Wall RR/LConn1 -- Contact Force Wall Body/LConn1 -- Contact Force Wall FL/LConn1 -- Contact Force Wall RL/LConn1 -- Contact Force Wall FR/LConn1 -- Conn5/RConn1
  Contact Force Wall FR/RConn1 -- FR/RConn1
  Contact Force Wall RL/RConn1 -- RL/RConn1
  Contact Force Wall RR/RConn1 -- RR/RConn1
  Contact Force Wall FL/RConn1 -- FL/RConn1
  Contact Force Wall Body/RConn1 -- Body/RConn1
  PS-Simulink Converter/LConn1 -- Contact Force Wall RR/RConn2
  Contact Force Wall FR/RConn2 -- PS-Simulink Converter1/LConn1
  Contact Force Wall FL/RConn2 -- PS-Simulink Converter3/LConn1
  Contact Force Wall RL/RConn2 -- PS-Simulink Converter2/LConn1
